simulink model "leftTurn_simulink1"  (Simulink 8.4)
settings: Solver=ode45  SolverMode=SingleTasking  StartTime=0.0  StopTime=10.0  RelTol=1e-3
values from neighbouring files (symbols this model uses):
  aAEB = -5.8    [ACCAEBIni.m]
  AbsAccMax = 3.5    [ACCAEBIni.m]
  AEBTTCInput = AEBTTCInputFun(SpdMinData_kmph,vAEBData_kmph,TTCAEBData,TTCAEBMax,Car_AEB)    [ACCAEBIni.m]    (also in AEBTTCInputFun.m = [kmph2mps([SpdMinData_kmph,40]);         [TTCAEBData(1)+(TTC)
  g = 9.8    [ACCAEBIni.m]
  HeadwayTime_desire = 1    [ACCAEBIni.m]
  Kpid = [Kp,Ki,Kd]    [ACCAEBIni.m]
  rAEB = -12    [ACCAEBIni.m]
  RoadFrictionCoeff = 0.8    [ACCAEBIni.m]
undefined symbols (not defined in the file or in its folder): hx0, hy0, lx0, ly0, nTest, RMin, StopWhenAEBOn, Ts, vIni
libraries: simulink x3
settings Model: Creator=zhaoding  LastModifiedBy=gyh  CovMetricSettings=dwe  CovHtmlReporting=off  covSaveCumulativeToWorkspaceVar=off  CovSaveSingleToWorkspaceVar=off  CovExternalEMLEnable=on  CovSFcnEnable=on
settings DataIOCC: LimitDataPoints=off  SaveFormat=StructureWithTime  SignalLoggingSaveFormat=Dataset
settings OptimizationCC: ExpressionDepthLimit=128
settings DebuggingCC: UnderspecifiedInitializationDetection=Simplified  MergeDetectMultiDrivingBlocksExec=error  SolverPrmCheckMsg=none  FcnCallInpInsideContextMsg=EnableAllAsError  FrameProcessingCompatibilityMsg=error  StateNameClashWarn=none  SFUnexpectedBacktrackingDiag=error  SFNoUnconditionalDefaultTransitionDiag=error
settings HardwareCC: ProdBitPerPointer=64  ProdLargestAtomicFloat=Float  ProdIntDivRoundTo=Zero  ProdEndianess=LittleEndian  ProdHWDeviceType=Specified
settings ModelReferenceCC: PropagateSignalLabelsOutOfModel=on
settings GRTTargetCC: TargetLangStandard=C99 (ISO)  GeneratePreprocessorConditionals=Use local settings  CombineOutputUpdateFcns=on  GRTInterface=off

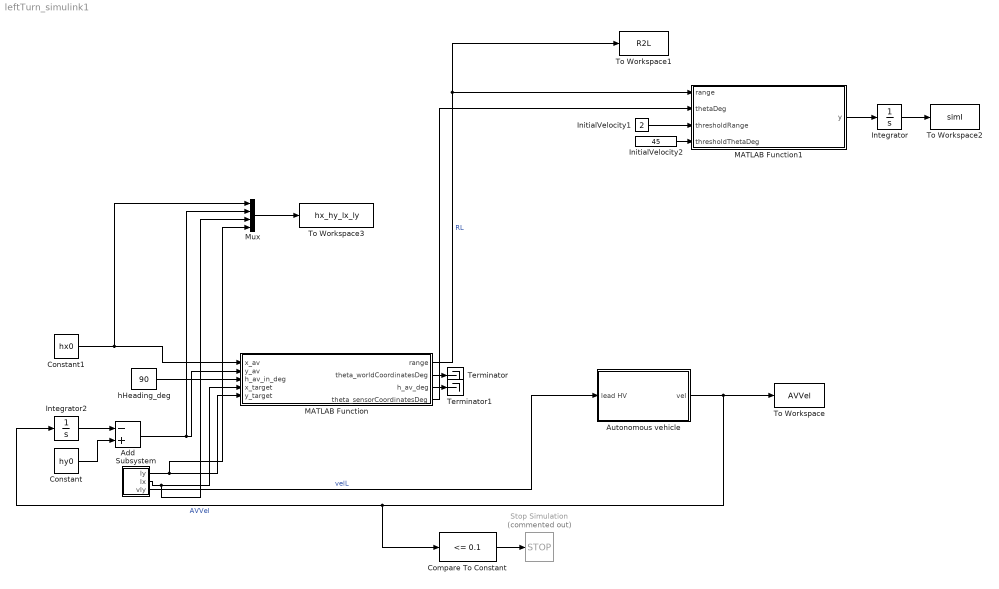
== system leftTurn_simulink1 ==
  Add : Sum  Inputs=-+
  Autonomous vehicle : Subsystem
  Compare To Constant : simulink/Logic and Bit Operations/Compare To Constant  relop=<=  const=0.1  OutDataTypeStr=boolean
  Constant : Constant  Value=hy0
  Constant1 : Constant  Value=hx0
  InitialVelocity1 : Constant  Tag=InitialVelocity  Value=2
  InitialVelocity2 : Constant  Tag=InitialVelocity  Value=45
  Integrator : Integrator
  Integrator2 : Integrator
  MATLAB Function : MATLAB Function  TreatAsAtomicUnit=on
      settings: PermitHierarchicalResolution=ParametersOnly
  MATLAB Function1 : MATLAB Function  TreatAsAtomicUnit=on
      settings: PermitHierarchicalResolution=ParametersOnly
  Mux : Mux
  Stop Simulation : Stop  Commented=on
  Subsystem : Subsystem
  Terminator : Terminator
  Terminator1 : Terminator
  To Workspace : ToWorkspace  VariableName=AVVel  SaveFormat=Timeseries  SampleTime=-1
  To Workspace1 : ToWorkspace  VariableName=R2L  SaveFormat=Timeseries  SampleTime=-1
  To Workspace2 : ToWorkspace  VariableName=simI  SaveFormat=Timeseries  SampleTime=-1
  To Workspace3 : ToWorkspace  VariableName=hx_hy_lx_ly  SaveFormat=Timeseries  SampleTime=-1
  hHeading_deg : Constant  Value=90
  wires:
  Subsystem/3(vly) -> Autonomous vehicle/1(lead HV)  "velL"
  Integrator2/1 -> Add/1
  Constant/1 -> Add/2
  Constant1/1 -> Mux/1, MATLAB Function/1(x_av)
  Add/1 -> Mux/2, MATLAB Function/2(y_av)
  hHeading_deg/1 -> MATLAB Function/3(h_av_in_deg)
  Subsystem/1(ly) -> Mux/4, MATLAB Function/5(y_target)
  Subsystem/2(lx) -> Mux/3, MATLAB Function/4(x_target)
  MATLAB Function/2(theta_worldCoordinatesDeg) -> Terminator/1
  MATLAB Function/3(h_av_deg) -> Terminator1/1
  InitialVelocity2/1 -> MATLAB Function1/4(thresholdThetaDeg)
  MATLAB Function/4(theta_sensorCoordinatesDeg) -> MATLAB Function1/2(thetaDeg)
  InitialVelocity1/1 -> MATLAB Function1/3(thresholdRange)
  MATLAB Function/1(range) -> To Workspace1/1, MATLAB Function1/1(range)  "RL"
  MATLAB Function1/1(y) -> Integrator/1
  Integrator/1 -> To Workspace2/1
  Mux/1 -> To Workspace3/1
  Autonomous vehicle/1(vel) -> Compare To Constant/1, Integrator2/1, To Workspace/1  "AVVel"
  Compare To Constant/1 -> Stop Simulation/1

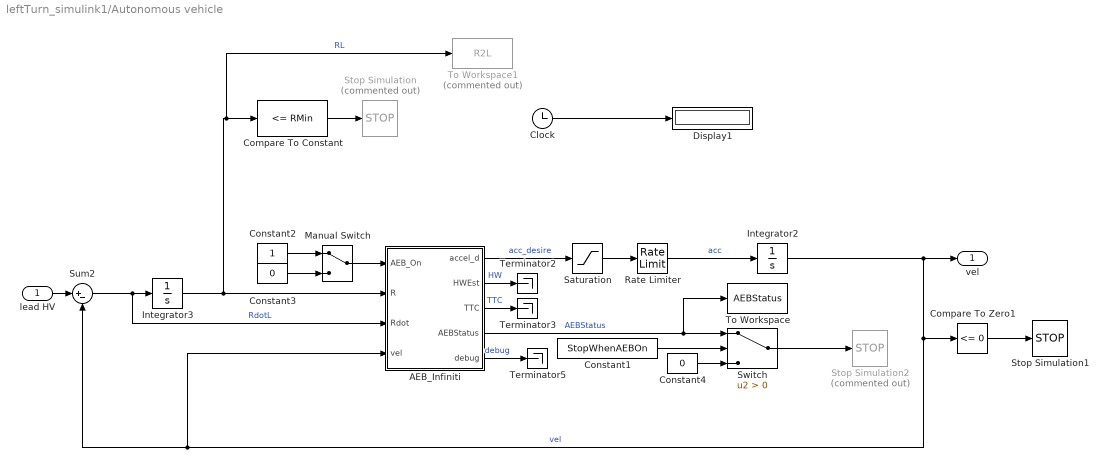
== system leftTurn_simulink1/Autonomous vehicle ==
  lead HV : Inport
  AEB_Infiniti : MATLAB Function  TreatAsAtomicUnit=on  SystemSampleTime=Ts
      settings: PermitHierarchicalResolution=ParametersOnly
  Clock : Clock
  Compare To Constant : simulink/Logic and Bit Operations/Compare To Constant  relop=<=  const=RMin  OutDataTypeStr=boolean
  Compare To Zero1 : simulink/Logic and Bit Operations/Compare To Zero  relop=<=  OutDataTypeStr=boolean
  Constant1 : Constant  Value=StopWhenAEBOn  SampleTime=Ts
  Constant2 : Constant  SampleTime=Ts
  Constant3 : Constant  Value=0  SampleTime=Ts
  Constant4 : Constant  Value=0  SampleTime=Ts
  Display1 : Display
  Integrator2 : Integrator  InitialCondition=vIni(nTest)  LowerSaturationLimit=0
  Integrator3 : Integrator  InitialCondition=abs(hy0 - ly0)
  Manual Switch : ManualSwitch
  Rate Limiter : RateLimiter  RisingSlewLimit=20  FallingSlewLimit=-20  SampleTimeMode=inherited
  Saturation : Saturate  UpperLimit=RoadFrictionCoeff*g  LowerLimit=-RoadFrictionCoeff*g
  Stop Simulation : Stop  Commented=on
  Stop Simulation1 : Stop
  Stop Simulation2 : Stop  Commented=on
  Sum2 : Sum  Inputs=|+-
  Switch : Switch  Criteria=u2 > Threshold
  Terminator2 : Terminator
  Terminator3 : Terminator
  Terminator5 : Terminator
  To Workspace : ToWorkspace  VariableName=AEBStatus  SaveFormat=Timeseries  SampleTime=-1
  To Workspace1 : ToWorkspace  Commented=on  VariableName=R2L  SaveFormat=Timeseries  SampleTime=-1
  vel : Outport
  wires:
  AEB_Infiniti/1(accel_d) -> Saturation/1  "acc_desire"
  Sum2/1 -> AEB_Infiniti/3(Rdot), Integrator3/1  "RdotL"
  Integrator3/1 -> To Workspace1/1, Compare To Constant/1, AEB_Infiniti/2(R)  "RL"
  Saturation/1 -> Rate Limiter/1
  Compare To Constant/1 -> Stop Simulation/1
  lead HV/1 -> Sum2/1
  AEB_Infiniti/2(HWEst) -> Terminator2/1  "HW"
  AEB_Infiniti/3(TTC) -> Terminator3/1  "TTC"
  Manual Switch/1 -> AEB_Infiniti/1(AEB_On)
  Constant2/1 -> Manual Switch/1
  Constant3/1 -> Manual Switch/2
  AEB_Infiniti/4(AEBStatus) -> Switch/1, To Workspace/1  "AEBStatus"
  AEB_Infiniti/5(debug) -> Terminator5/1  "debug"
  Clock/1 -> Display1/1
  Integrator2/1 -> AEB_Infiniti/4(vel), Sum2/2, Compare To Zero1/1, vel/1  "vel"
  Compare To Zero1/1 -> Stop Simulation1/1
  Rate Limiter/1 -> Integrator2/1  "acc"
  Switch/1 -> Stop Simulation2/1
  Constant1/1 -> Switch/2
  Constant4/1 -> Switch/3

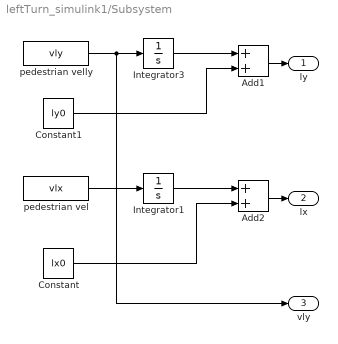
== system leftTurn_simulink1/Subsystem ==
  Add1 : Sum
  Add2 : Sum
  Constant : Constant  Value=lx0
  Constant1 : Constant  Value=ly0
  Integrator1 : Integrator
  Integrator3 : Integrator
  pedestrian vel : FromWorkspace  VariableName=vlx  SampleTime=0
  pedestrian velly : FromWorkspace  VariableName=vly  SampleTime=0
  ly : Outport
  lx : Outport  Port=2
  vly : Outport  Port=3
  wires:
  Integrator3/1 -> Add1/1
  Constant1/1 -> Add1/2
  pedestrian velly/1 -> vly/1, Integrator3/1
  Add1/1 -> ly/1
  Constant/1 -> Add2/2
  Add2/1 -> lx/1
  pedestrian vel/1 -> Integrator1/1
  Integrator1/1 -> Add2/1

== matlab function MATLAB Function1 ==
  data: range input double; y output double; thetaDeg input double; thresholdRange input double; thresholdThetaDeg input double
function y = fcn(range,thetaDeg,thresholdRange,thresholdThetaDeg)

if range < thresholdRange && abs(thetaDeg)<thresholdThetaDeg
    y = 1;
elseif range < 2.1
    y = 1;
else
    y = 0;
end
end

== matlab function Autonomous vehicle/AEB_Infiniti ==
  data: AEB_On input double; HeadwayTime_desire parameter double; R input double; Rdot input double; accel_d output double; vel input double; Kpid parameter double; HWEst output double; TTC output double; AEBStatus output double; debug output double; rAEB parameter double; aAEB parameter double; AEBTTCInput parameter double; AbsAccMax parameter double
function [accel_d,HWEst,TTC,AEBStatus,debug] = fcn(AEB_On, HeadwayTime_desire,R,Rdot,vel,Kpid,rAEB,aAEB,AEBTTCInput,AbsAccMax)
%#codegen
persistent HWErr AEBFlag accLog AEBTimer AEBIniAcc
if isempty(HWErr), HWErr = 0;end;
if isempty(AEBFlag), AEBFlag = 0;end;
if isempty(accLog), accLog = 0;end;
if isempty(AEBTimer), AEBTimer = 0;end;
if isempty(AEBIniAcc), AEBIniAcc = 0;end;
HWErrLast = HWErr;
AEBFlagLast = AEBFlag;
Ts = 0.1; % sampling time
HW_d = HeadwayTime_desire;
%% ACC setting
HWEst = R/vel;
HWErr = HW_d - HWEst;
Kp = Kpid(1);
Ki = Kpid(2);
% Kd = Kpid(3);
accMax = AbsAccMax;
accMin = -AbsAccMax;

%% AEB setting
% VelLead = Rdot-vel; Rdot-vel
TTC = -R/Rdot;
TTC_AEBRelease = 1;


%% AEB trigger
% AEBTTCInput = [    4.1667   11.1111;
%                    0.8579    0.9100;
%                    0.0075         0];

if isempty(find(AEBTTCInput(1,:)<=vel,1,'last'))
%     fprintf('PieceInd is empty');
    PieceInd= 1;
else
    PieceInd = min(find(AEBTTCInput(1,:)<=vel,1,'last'));
end
    
TTC_AEB = AEBTTCInput(2,PieceInd)+AEBTTCInput(3,PieceInd)*(vel-AEBTTCInput(1,PieceInd));
% if isempty(PieceInd)
%     fprintf('PieceInd is empty');
%     PieceInd= 1;
% end
if TTC > 0 && TTC <= TTC_AEB && AEB_On == 1
    AEBFlag = 1;
elseif TTC > TTC_AEBRelease || TTC < 0
    AEBFlag = 0;
end
debug = [AEBFlagLast;AEBFlag;HWErrLast];
AEBStatus = AEBFlag;
%% control
if AEBFlag == 0
    if AEBFlagLast == 1
        HWErrLast = 0;
        AEBTimer = 0;
    end
    accel_d = accLog+Kp*(HWErr-HWErrLast)+Ki*Ts/2*(HWErr+HWErrLast); % pi controller
    if vel >= 90/2.236 && accel_d > 0 % 70 mph speed limit
        accel_d = 0;
    else
        accel_d = max(min(accel_d,accMax),accMin);
    end
else
    if AEBFlagLast == 0
        AEBIniAcc = accLog;
    end
    AEBTimer = AEBTimer + 0.1;
    accel_d = AEBIniAcc + AEBTimer*rAEB;
    accel_d = max(aAEB,accel_d);
%     debug = [0,0,0];
end
accLog = accel_d;

== matlab function MATLAB Function ==
  data: x_av input double; range output double; y_av input double; h_av_in_deg input double; x_target input double; y_target input double; theta_worldCoordinatesDeg output double; h_av_deg output double; theta_sensorCoordinatesDeg output double
function [range,theta_worldCoordinatesDeg,h_av_deg,theta_sensorCoordinatesDeg] = fcn(x_av,y_av,h_av_in_deg,x_target,y_target)
    
    range = norm([x_av-x_target,y_av-y_target]);
    theta_worldCoordinatesDeg = atan2(x_target-x_av,y_target-y_av)*180/pi;
    h_av_deg = h_av_in_deg;
    theta_sensorCoordinatesDeg = ((theta_worldCoordinatesDeg-h_av_deg)*pi/180);
    theta_sensorCoordinatesDeg = mod(theta_sensorCoordinatesDeg + pi,2*pi) - pi;
    theta_sensorCoordinatesDeg = theta_sensorCoordinatesDeg/pi*180;
end
